simulink model "Ejemplo1"  (R2023a)
settings: Solver=VariableStepAuto  StartTime=0.0  StopTime=10.0  RelTol=1e-3
settings Model: Creator=mluser  LastModifiedBy=mluser

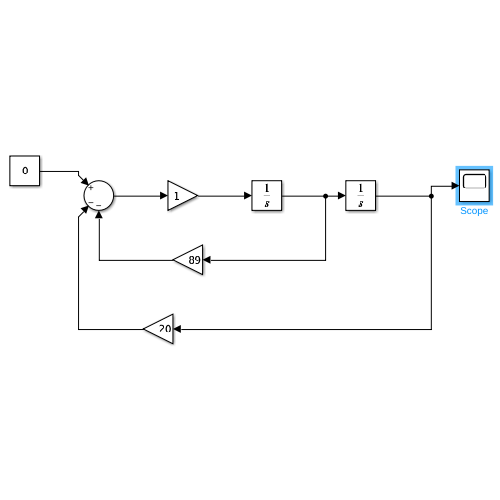
[thumbnail: Simulink's stored preview of the top-level diagram]
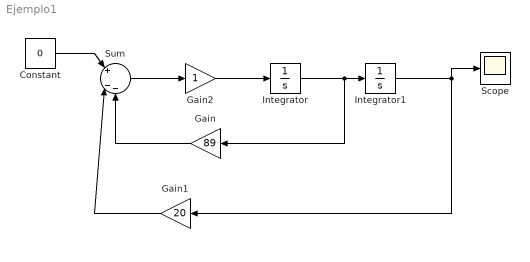
== system Ejemplo1 ==
  Constant : Constant  Value=0
  Gain : Gain  Gain=89
  Gain1 : Gain  Gain=20
  Gain2 : Gain
  Integrator : Integrator
  Integrator1 : Integrator  InitialCondition=0.5
  Scope : Scope
  Sum : Sum  Inputs=|+|--
  wires:
  Integrator/1 -> Gain/1, Integrator1/1
  Constant/1 -> Sum/1
  Gain/1 -> Sum/3
  Integrator1/1 -> Scope/1, Gain1/1
  Gain1/1 -> Sum/2
  Gain2/1 -> Integrator/1
  Sum/1 -> Gain2/1
